simulink model "task4_model"  (R2018a)
settings: Solver=VariableStepAuto  StartTime=0.0  StopTime=20  RelTol=1e-3
values from neighbouring files (symbols this model uses):
  A = [-8.8487+(a-b)/5, -0.0399, -5.55+(c+d)/10, 3.5846 ... (first row only)    [task1.m]    (also in task2.m; task3.m; task4.m; task5.m)
  B = [0.0564+b/(10+c), 0.0319 ... (first row only)    [task1.m]    (also in task2.m; task3.m; task4.m; task5.m)
  C = [-3.2988,-2.1932+(10*c+d)/(100+5*a), 0.0370, -0.0109 ... (first row only)    [task1.m]    (also in task2.m; task3.m; task4.m; task5.m)
  F = inv(C*(inv(-A+B*K))*B)    [task2.m]    (also in task4.m = inv(Bstar); task5.m = round(inv(Cbar*(inv(-Abar+Bbar*K))*Bbar),4))
  K = Kbar*T    [task1.m]    (also in task2.m = round(((inv(R))*(transpose(B))*P),4); task3.m = round(((inv(R))*(transpose(B))*P),4); task4.m = (inv(Bstar))*Cstarstar; task5.m = round(((inv(R))*(transpose(Bbar))*P),4))
  X0 = [0.5;-0.1;0.3;-0.8]    [task1.m]    (also in task2.m; task3.m; task4.m; task5.m)
settings Model: Creator=PYT  LastModifiedBy=PYT

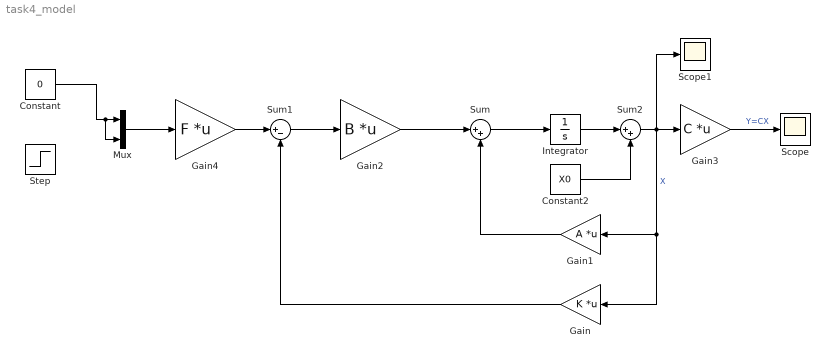
== system task4_model ==
  Constant : Constant  Value=0
  Constant2 : Constant  Value=X0
  Gain : Gain  Gain=K  Multiplication=Matrix(K*u)
  Gain1 : Gain  Gain=A  Multiplication=Matrix(K*u)
  Gain2 : Gain  Gain=B  Multiplication=Matrix(K*u)
  Gain3 : Gain  Gain=C  Multiplication=Matrix(K*u)
  Gain4 : Gain  Gain=F  Multiplication=Matrix(K*u)
  Integrator : Integrator
  Mux : Mux  Inputs=2
  Scope : Scope
  Scope1 : Scope
  Step : Step  Time=0  SampleTime=0
  Sum : Sum  Inputs=|++
  Sum1 : Sum  Inputs=|+-
  Sum2 : Sum  Inputs=|++
  wires:
  Sum/1 -> Integrator/1
  Gain1/1 -> Sum/2
  Gain2/1 -> Sum/1
  Sum1/1 -> Gain2/1
  Gain/1 -> Sum1/2
  Mux/1 -> Gain4/1
  Gain3/1 -> Scope/1  "Y=CX"
  Constant/1 -> Mux/1, Mux/2
  Gain4/1 -> Sum1/1
  Integrator/1 -> Sum2/1
  Sum2/1 -> Scope1/1, Gain/1, Gain1/1, Gain3/1  "X"
  Constant2/1 -> Sum2/2
